simulink model "lab33"  (R2023a)
settings: Solver=VariableStepAuto  StartTime=0.0  StopTime=50  MaxStep=0.02  RelTol=1e-3
settings Model: Creator=wendy  LastModifiedBy=wendy

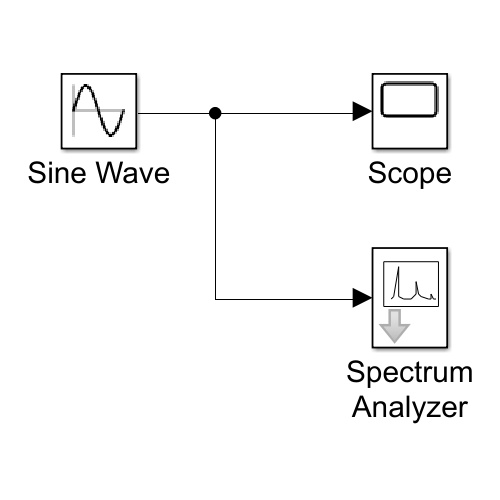
[thumbnail: Simulink's stored preview of the top-level diagram]
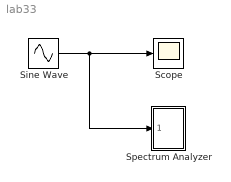
== system lab33 ==
  Scope : Scope
  Sine Wave : Sin  Frequency=5*pi  SampleTime=0
  Spectrum Analyzer : Subsystem  mask(Spectrum analyzer.){N=2048, T_s=0.02, plot_period=10}
      mask prompts: N "Number of sample points:"; T_s "Sampling period (sec):"; plot_period "Plotting Period (sec):"
      mask Help: EE438 Lab utility; See Prof. Bouman.
      mask Display: plot(0,0,100,100,[14,91,91,14,14],[86,86,40,40,86],[85,82,80,79,75,67,63,60,57,53,41,36,33,27,24],[49,50,53,50,49,51,54,66,54,50,50,52,81,51,49])
  wires:
  Sine Wave/1 -> Spectrum Analyzer/1(input signal), Scope/1

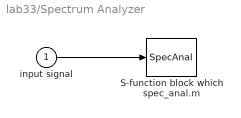
== system lab33/Spectrum Analyzer ==
  input signal : Inport
  S-function block which spec_anal.m : S-Function  FunctionName=SpecAnal  Parameters=N,T_s,plot_period  SFunctionDeploymentMode=off  EnableBusSupport=off
  wires:
  input signal/1 -> S-function block which spec_anal.m/1
